simulink model "pid_shirato"  (R2020a)
settings: Solver=VariableStepAuto  StartTime=0.0  StopTime=2.0  RelTol=1e-3
libraries: cstblocks x2
settings Model: Creator=yuimu  LastModifiedBy=yuimu
settings SFSimCC: CustomCodeUndefinedFunction=UseInterfaceOnly

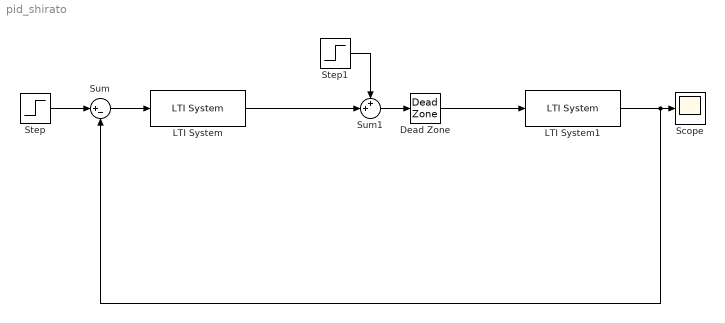
== system pid_shirato ==
  Dead Zone : DeadZone  LowerValue=-0.8  UpperValue=0.8  SaturateOnIntegerOverflow=on
  LTI System : cstblocks/LTI System  sys=Cpid  IC=[]
  LTI System1 : cstblocks/LTI System  sys=Gnominal  IC=[]
  Scope : Scope
  Step : Step  Time=0  After=5  SampleTime=0
  Step1 : Step  After=0  SampleTime=0
  Sum : Sum  Inputs=|+-
  Sum1 : Sum  Inputs=++|
  wires:
  Step1/1 -> Sum1/1
  Sum1/1 -> Dead Zone/1
  Step/1 -> Sum/1
  LTI System1/1 -> Sum/2, Scope/1
  Sum/1 -> LTI System/1
  LTI System/1 -> Sum1/2
  Dead Zone/1 -> LTI System1/1
